simulink model "Problem8"  (R2020b)
settings: Solver=VariableStepAuto  StartTime=0.0  StopTime=inf  RelTol=1e-3
settings Model: PacingRate=0.028000  Creator=vigne  LastModifiedBy=Hp

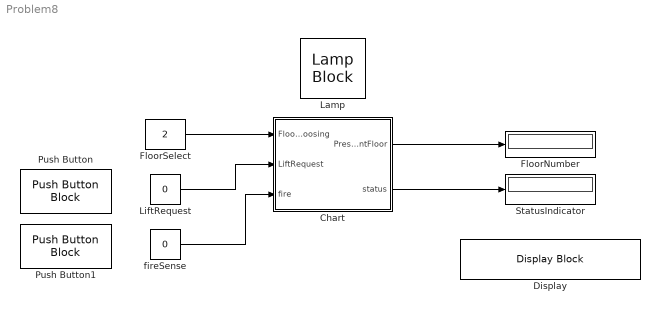
== system Problem8 ==
  Chart : Stateflow chart  TreatAsAtomicUnit=on
  Display : DisplayBlock  LabelPosition=Hide  Format=short  Transparency=1
  FloorNumber : Display
  FloorSelect : Constant  Value=2
  Lamp : LampBlock
  LiftRequest : Constant  Value=0
  Push Button : PushButtonBlock
  Push Button1 : PushButtonBlock
  StatusIndicator : Display
  fireSense : Constant  Value=0
  wires:
  FloorSelect/1 -> Chart/1(Floorchoosing)
  LiftRequest/1 -> Chart/2(LiftRequest)
  fireSense/1 -> Chart/3(fire)
  Chart/1(PresentFloor) -> FloorNumber/1
  Chart/2(status) -> StatusIndicator/1

== stateflow chart Problem8/Chart ==
  state LiftOperation [parallel]
    entry:
    status=0;
    settings: executionOrder=1
    state LiftFunctionOn
      state FifthFloor
        entry:
        status=1;
        during:
        PresentFloor=5;
        Floorchecking(PresentFloor);
        exit:
        status=0;
      state GroundFloor
        entry:
        status=1;
        during:
        PresentFloor=0;
        Floorchecking(PresentFloor);
        exit:
        status=0;
        (history)
      state FourthFloor
        entry:
        status=1
        during:
        PresentFloor=4;
        Floorchecking(PresentFloor);
        exit:
        status=0;
      state FirstFloor
        entry:
        status=1;
        during:
        PresentFloor=1;
        Floorchecking(PresentFloor);
        exit:
        status=0;
      state SecondFloor
        entry:
        status=1;
        during:
        PresentFloor=2;
        Floorchecking(PresentFloor);
        exit:
        status=0;
        after(1,sec);
      state ThirdFloor
        entry:
        status=1;
        during:
        PresentFloor=3;
        Floorchecking(PresentFloor);
        exit:
        status=0;
        after(1,sec);
      (default) -> GroundFloor
      FourthFloor -> FifthFloor [order 2] : up
      FifthFloor -> FourthFloor : down
      GroundFloor -> FirstFloor : up
      FirstFloor -> GroundFloor [order 2] : down
      FirstFloor -> SecondFloor [order 1] : up
      SecondFloor -> FirstFloor [order 2] : down
      FourthFloor -> ThirdFloor [order 1] : down
      ThirdFloor -> FourthFloor [order 1] : up
      SecondFloor -> ThirdFloor [order 1] : up
      ThirdFloor -> SecondFloor [order 2] : down
    state LiftFunctionOff
      en:
      status=0;
    (default) -> LiftFunctionOn
    LiftFunctionOff -> LiftFunctionOn : [fire==0]
    LiftFunctionOn -> LiftFunctionOff : [fire==1]
  state y = Floorchecking(Floor) [function]
    (default) -> (junction 62)
    (junction 62) -> (junction 71) [order 3] : [Floorchoosing<Floor]{
        | send(down);
        | disp('LiftMovingDown');}
    (junction 62) -> (junction 65) [order 1] : [Floorchoosing>Floor]{
        | send(up);
        | disp('LiftMovingUp');}
    (junction 62) -> (junction 67) [order 2] : [Floorchoosing==Floor]{
        | disp('CurrentFloor');}
    (junction 71) -> (junction 86)
    (junction 65) -> (junction 89)
    (junction 86) -> (junction 67)
    (junction 89) -> (junction 67)
    (junction 67) -> (junction 69)
  data: Floor function_input; y function_output; Floorchoosing input; LiftRequest input; PresentFloor output; status output; fire input; alarmStatus local
  events: up local FUNCTION_CALL_EVENT; down local FUNCTION_CALL_EVENT
